simulink model "Tisch"  (R2017b)
settings: Solver=VariableStepAuto  StartTime=0.0  StopTime=10.0  RelTol=1e-3
settings Model: Creator=aby032  LastModifiedBy=aby032

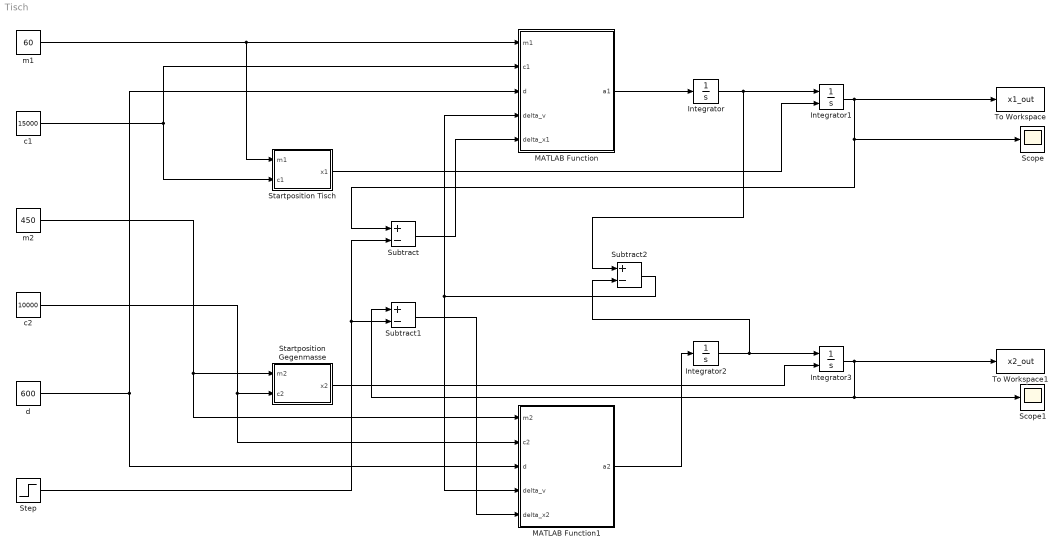
== system Tisch ==
  Integrator : Integrator
  Integrator1 : Integrator  InitialConditionSource=external
  Integrator2 : Integrator
  Integrator3 : Integrator  InitialConditionSource=external
  MATLAB Function : MATLAB Function  TreatAsAtomicUnit=on
  MATLAB Function1 : MATLAB Function  TreatAsAtomicUnit=on
  Scope : Scope
  Scope1 : Scope
  Startposition Gegenmasse : MATLAB Function  TreatAsAtomicUnit=on
  Startposition Tisch : MATLAB Function  TreatAsAtomicUnit=on
  Step : Step  Time=0.5  After=0.001  SampleTime=0
  Subtract : Sum  Inputs=+-
  Subtract1 : Sum  Inputs=+-
  Subtract2 : Sum  Inputs=+-
  To Workspace : ToWorkspace  VariableName=x1_out  SaveFormat=Timeseries  SampleTime=-1
  To Workspace1 : ToWorkspace  VariableName=x2_out  SaveFormat=Timeseries  SampleTime=-1
  c1 : Constant  Value=15000
  c2 : Constant  Value=10000
  d : Constant  Value=600
  "m1 " : Constant  Value=60
  m2 : Constant  Value=450
  wires:
  "m1 "/1 -> Startposition Tisch/1(m1), MATLAB Function/1(m1)
  c1/1 -> MATLAB Function/2(c1), Startposition Tisch/2(c1)
  m2/1 -> Startposition Gegenmasse/1(m2), MATLAB Function1/1(m2)
  c2/1 -> Startposition Gegenmasse/2(c2), MATLAB Function1/2(c2)
  d/1 -> MATLAB Function/3(d), MATLAB Function1/3(d)
  MATLAB Function/1(a1) -> Integrator/1
  MATLAB Function1/1(a2) -> Integrator2/1
  Integrator2/1 -> Subtract2/2, Integrator3/1
  Integrator/1 -> Subtract2/1, Integrator1/1
  Startposition Gegenmasse/1(x2) -> Integrator3/2
  Startposition Tisch/1(x1) -> Integrator1/2
  Step/1 -> Subtract/2, Subtract1/2
  Integrator1/1 -> Subtract/1, Scope/1, To Workspace/1
  Integrator3/1 -> Scope1/1, Subtract1/1, To Workspace1/1
  Subtract1/1 -> MATLAB Function1/5(delta_x2)
  Subtract/1 -> MATLAB Function/5(delta_x1)
  Subtract2/1 -> MATLAB Function1/4(delta_v), MATLAB Function/4(delta_v)

== matlab function Tisch/Startposition Gegenmasse ==
  data: m2 input; c2 input; x2 output
function x2 = fcn(m2,c2)
g = 9.80665;                    %Erdbeschleunigung
x2 = -(m2*g)/(2*c2);

== matlab function Tisch/Startposition Tisch ==
  data: m1 input; c1 input; x1 output
function x1 = fcn(m1,c1)
g = 9.80665;                    %Erdbeschleunigung
x1 = -(m1*g)/(2*c1);

== matlab function Tisch/MATLAB Function ==
  data: m1 input; a1 output; c1 input; d input; delta_v input; delta_x1 input
function a1 = fcn(m1,c1,d,delta_v,delta_x1)
g = 9.80665;                    %Erdbeschleunigung

Fg1 = m1*g;                     %Kraft Tisch
Fc1 = 2*c1*delta_x1;            %Kraft Feder 1
Fd = 2*d*delta_v;


a1 = (-Fg1-Fc1-Fd)/m1;

== matlab function Tisch/MATLAB Function1 ==
  data: m2 input; a2 output; c2 input; d input; delta_v input; delta_x2 input
function a2 = fcn(m2,c2,d,delta_v,delta_x2)
g = 9.80665;                    %Erdbeschleunigung

Fg2 = m2*g;                     %Kraft Gegenmasse
Fc2 = 2*c2*delta_x2;            %Kraft  Feder 2
Fd = 2*d*delta_v;


a2 = (-Fg2-Fc2+Fd)/m2;
